simulink model "transmisorUSRP"  (R2025b)
settings: Solver=FixedStepDiscrete  StartTime=0.0  StopTime=7000  FixedStep=1/3312  RelTol=1e-3
libraries: commcnvcod2 x1, commsdrhw_v2 x1, commdigbbndpm3 x1, commfilt2 x1
settings Model: VariantFading=off  Creator=karolpalechor  LastModifiedBy=briyi

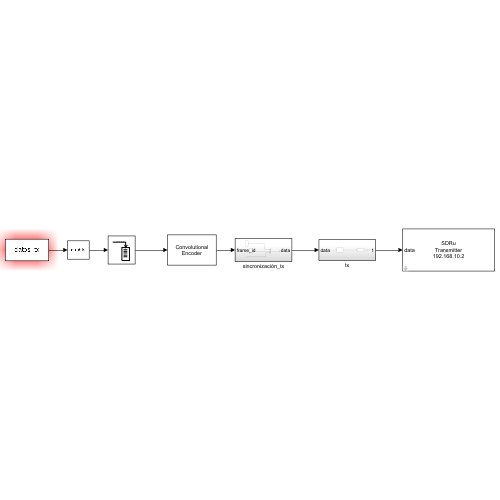
[thumbnail: Simulink's stored preview of the top-level diagram]
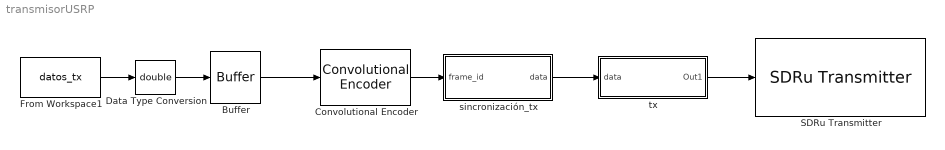
== system transmisorUSRP ==
  Buffer : Buffer  N=1656  OutputFrames=off
  Convolutional Encoder : commcnvcod2/Convolutional Encoder  trellis=poly2trellis(7, [171 133])  opMode=Continuous  DelayedResetAction=off  hasIniStPort=off  hasFinStPort=off  usePuncVector=off  punctureVector=[1; 1; 0; 1; 0; 1]  reset=Unused parameter value
  Data Type Conversion : DataTypeConversion  OutDataTypeStr=double  SaturateOnIntegerOverflow=off  RndMeth=Floor
  From Workspace1 : FromWorkspace  VariableName=datos_tx  OutDataTypeStr=uint8  SampleTime=1/1656  Interpolate=off  ZeroCross=off  OutputAfterFinalValue=Holding final value
  SDRu Transmitter : commsdrhw_v2/SDRu Transmitter  rxtx=tx  initializeIPAddress=0  devMap=0  USRP2_IP=192.168.10.2  USRP_IP_X300=192.168.10.2  USRP_IP_X310=192.168.10.2  USRP_IP_N300=No devices found  USRP_IP_N310=192.168.10.2  USRP_IP_N320=No devices found  USRP_IP_E320=No devices found  USRP_IP_X410=No devices found  USRP_serialNumB200=3136D21  USRP_serialNumB210=No devices found  platform=N200/N210/USRP2  prevPlatform=N200/N210/USRP2  lastIPAddressPopup=192.168.10.2  USRP_ID=192.168.10.2  LastIPAddress=192.168.10.2  ChannelMapping=1  centerFrequencySrc=Dialog  centerFrequency=2.45e9  loOffsetSrc=Dialog  loOffset=0  gainSrc=Dialog  gain=8  PPSSource=Internal  clockSource=Internal  EnableGPSLock=off  EnsureSyncGPSTime=off  EnableTimeTrigger=off  triggerTime=5  enableMIMOCableSync=off  EnableRefLock=off  masterClkRateParam=100e6  masterClkRateB200=32e6  masterClkRateB210=32e6  masterClkRateX300=200e6  masterClkRateX310=200e6  masterClkRateN300=125e6  masterClkRateN310=125e6  masterClkRateN320=200e6  masterClkRateE320=30.72e6  masterClkRateX410=250e6  decimInterpSrc=Dialog  lastDecimSource=Dialog  decimInterp=512  USRP2_IP_NUM=[49 57 50 46 49 54 56 46 49 48 46 50]  frameLength=362  sampleRate=195312.5  TransportDataType=int16  outputDatatype=Same as transport data type  overrunUnderrunPort=off  sampleTime=5.12e-06  dboardInfo=|  HOST_DATA_PORT=30000  HOST_CONTROL_PORT=30001  USRP2_DATA_PORT=32769  USRP2_CONTROL_PORT=32768  bufferMode=Continuous streaming  EnableBurstMode=off  NumFramesInBurst=100
      | dbid: 0
      |           dbName: 'no db found'
      |          freqMin: 0
      |          freqMax: 0
      |          gainMin: 0
      |          gainMax: 0
      |     gainStepSize: 0
  sincronización_tx : Subsystem
  tx : Subsystem
  wires:
  From Workspace1/1 -> Data Type Conversion/1
  Data Type Conversion/1 -> Buffer/1
  Convolutional Encoder/1 -> sincronización_tx/1(frame_id)
  Buffer/1 -> Convolutional Encoder/1
  sincronización_tx/1(data) -> tx/1(data)
  tx/1(Out1) -> SDRu Transmitter/1

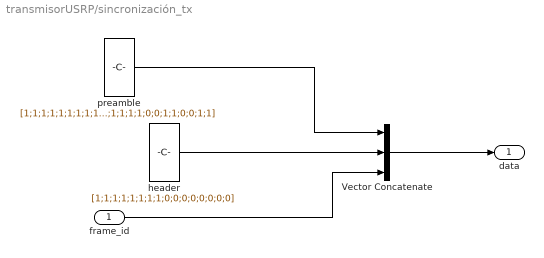
== system transmisorUSRP/sincronización_tx ==
  frame_id : Inport
  Vector Concatenate : Concatenate  NumInputs=3
  header : Constant  Value=[1;1;1;1;1;1;1;1;0;0;0;0;0;0;0;0]  VectorParams1D=off  OutDataTypeStr=double  SampleTime=-1
  preamble : Constant  Value=[1;1;1;1;1;1;1;1;1;1;0;0;0;0;1;1;1;1;0;0;1;1;0;0;1;1]  VectorParams1D=off  OutDataTypeStr=double  SampleTime=-1
  data : Outport
  wires:
  Vector Concatenate/1 -> data/1
  preamble/1 -> Vector Concatenate/1
  frame_id/1 -> Vector Concatenate/3
  header/1 -> Vector Concatenate/2

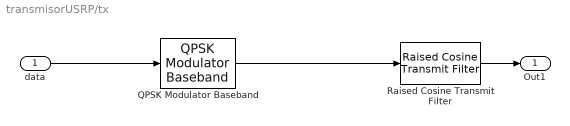
== system transmisorUSRP/tx ==
  data : Inport
  QPSK Modulator Baseband : commdigbbndpm3/QPSK Modulator Baseband  InType=Bit  Enc=Gray  Ph=pi/4  outDtype=Inherit via back propagation  outWordLen=16  outUDDataType=sfix(16)  outFracLenMode=Best precision  outFracLen=15  outDataTypeStr=Inherit: Inherit via back propagation  outLastDataTypeStr=Inherit: Inherit via back propagation
  Raised Cosine Transmit Filter : commfilt2/Raised Cosine Transmit Filter  filtType=Square root  R=0.25  filtSpan=10  N=8  filterGain=1  InputProcessing=Columns as channels (frame based)  RateOptions=Enforce single-rate processing  framing=Mute  checkCoeff=off  variableName=rcTxFilt  checkGain=Normalized  sampMode=Mute  saveAsFlag=0  currentFiltSpan=10  D=(10)/2  launchFVT=on  roundingMode=Floor  overflowMode=off  coeffDataTypeStr=Inherit: Same word length as input  coeffMin=[]  coeffMax=[]  coeffLastDataTypeStr=Inherit: Same word length as input  outputDataTypeStr=Inherit: Same as accumulator  outputMin=[]  outputMax=[]  outputLastDataTypeStr=Inherit: Same as accumulator
  Out1 : Outport
  wires:
  QPSK Modulator Baseband/1 -> Raised Cosine Transmit Filter/1
  Raised Cosine Transmit Filter/1 -> Out1/1
  data/1 -> QPSK Modulator Baseband/1
